simulink model "shr26df_user_input"  (R2024b)
settings: Solver=VariableStepAuto  StartTime=0.0  StopTime=10  RelTol=1e-3
undefined symbols (not defined in the file): X, Y, Z
libraries: sm_lib x261, nesl_utility x53
(part 1 of 6)
settings Model: Creator=danie  LastModifiedBy=danie

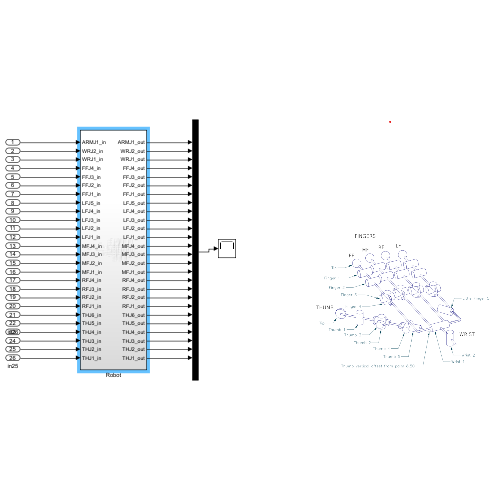
[thumbnail: Simulink's stored preview of the top-level diagram]
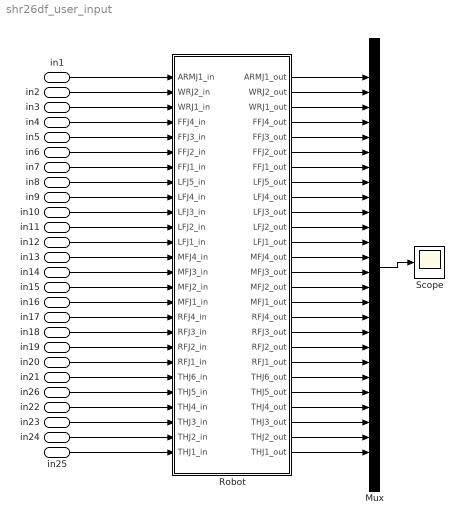
== system shr26df_user_input ==
  in1 : Inport
  in2 : Inport  Port=2
  in3 : Inport  Port=3
  in4 : Inport  Port=4
  in5 : Inport  Port=5
  in6 : Inport  Port=6
  in7 : Inport  Port=7
  in8 : Inport  Port=8
  in9 : Inport  Port=9
  in10 : Inport  Port=10
  in11 : Inport  Port=11
  in12 : Inport  Port=12
  in13 : Inport  Port=13
  in14 : Inport  Port=14
  in15 : Inport  Port=15
  in16 : Inport  Port=16
  in17 : Inport  Port=17
  in18 : Inport  Port=18
  in19 : Inport  Port=19
  in20 : Inport  Port=20
  in21 : Inport  Port=21
  in26 : Inport  Port=22
  in22 : Inport  Port=23
  in23 : Inport  Port=24
  in24 : Inport  Port=25
  in25 : Inport  Port=26
  Mux : Mux  Inputs=26
  Robot : Subsystem
  Scope : Scope
  wires:
  Mux/1 -> Scope/1
  Robot/1(ARMJ1_out) -> Mux/1
  Robot/2(WRJ2_out) -> Mux/2
  Robot/3(WRJ1_out) -> Mux/3
  Robot/4(FFJ4_out) -> Mux/4
  Robot/5(FFJ3_out) -> Mux/5
  Robot/6(FFJ2_out) -> Mux/6
  Robot/7(FFJ1_out) -> Mux/7
  Robot/8(LFJ5_out) -> Mux/8
  Robot/9(LFJ4_out) -> Mux/9
  Robot/10(LFJ3_out) -> Mux/10
  Robot/11(LFJ2_out) -> Mux/11
  Robot/12(LFJ1_out) -> Mux/12
  Robot/13(MFJ4_out) -> Mux/13
  Robot/14(MFJ3_out) -> Mux/14
  Robot/15(MFJ2_out) -> Mux/15
  Robot/16(MFJ1_out) -> Mux/16
  Robot/17(RFJ4_out) -> Mux/17
  Robot/18(RFJ3_out) -> Mux/18
  Robot/19(RFJ2_out) -> Mux/19
  Robot/20(RFJ1_out) -> Mux/20
  Robot/21(THJ6_out) -> Mux/21
  in1/1 -> Robot/1(ARMJ1_in)
  in2/1 -> Robot/2(WRJ2_in)
  in3/1 -> Robot/3(WRJ1_in)
  in4/1 -> Robot/4(FFJ4_in)
  in5/1 -> Robot/5(FFJ3_in)
  in6/1 -> Robot/6(FFJ2_in)
  in7/1 -> Robot/7(FFJ1_in)
  in8/1 -> Robot/8(LFJ5_in)
  in9/1 -> Robot/9(LFJ4_in)
  in10/1 -> Robot/10(LFJ3_in)
  in11/1 -> Robot/11(LFJ2_in)
  in12/1 -> Robot/12(LFJ1_in)
  in13/1 -> Robot/13(MFJ4_in)
  in14/1 -> Robot/14(MFJ3_in)
  in15/1 -> Robot/15(MFJ2_in)
  in16/1 -> Robot/16(MFJ1_in)
  in17/1 -> Robot/17(RFJ4_in)
  in18/1 -> Robot/18(RFJ3_in)
  in19/1 -> Robot/19(RFJ2_in)
  in20/1 -> Robot/20(RFJ1_in)
  in21/1 -> Robot/21(THJ6_in)
  in22/1 -> Robot/23(THJ4_in)
  in23/1 -> Robot/24(THJ3_in)
  in24/1 -> Robot/25(THJ2_in)
  in25/1 -> Robot/26(THJ1_in)
  Robot/22(THJ5_out) -> Mux/22
  Robot/23(THJ4_out) -> Mux/23
  Robot/24(THJ3_out) -> Mux/24
  Robot/25(THJ2_out) -> Mux/25
  Robot/26(THJ1_out) -> Mux/26
  in26/1 -> Robot/22(THJ5_in)
